simulink model "sensorExpoler_Lab1_1"  (R2026a)
settings: Solver=FixedStepAuto  StopTime=10  FixedStep=0.001
undefined symbols (not defined in the file or in its folder): Blocking, Non
libraries: amg_usbconverter_n_connect_lib x2
settings Model: Creator=pboon  LastModifiedBy=Kawpaan

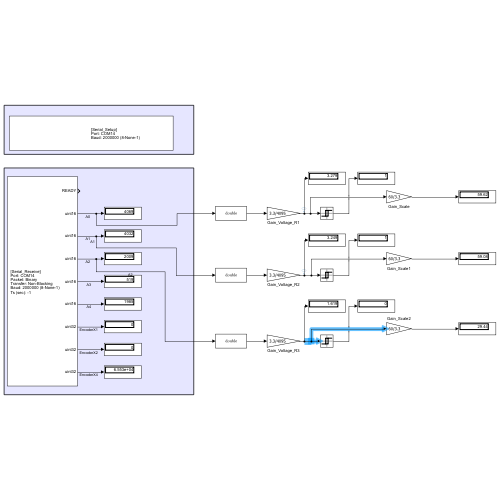
[thumbnail: Simulink's stored preview of the top-level diagram]
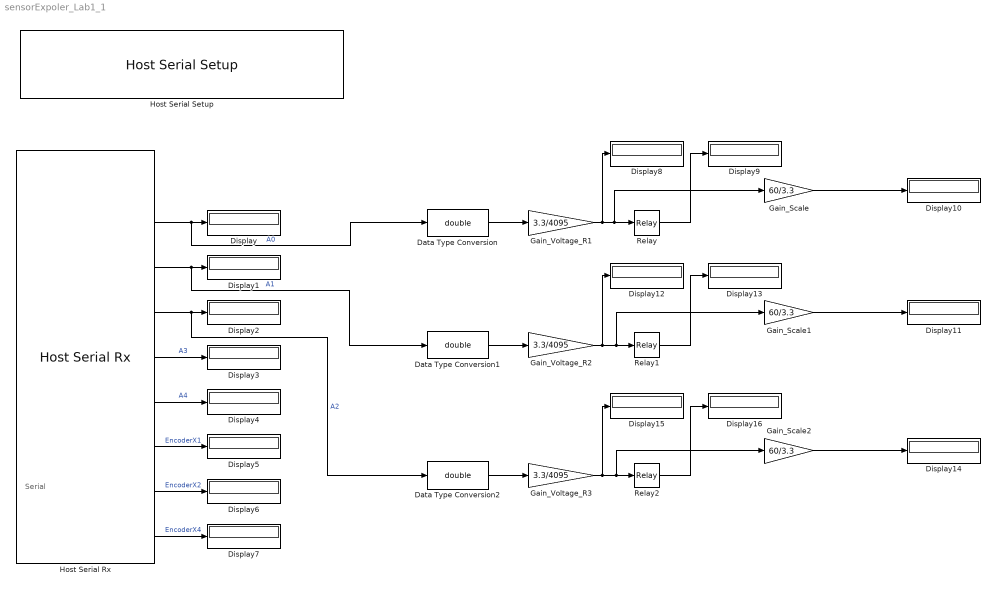
== system sensorExpoler_Lab1_1 ==
  note: Serial
  Data Type Conversion : DataTypeConversion  OutDataTypeStr=double  SaturateOnIntegerOverflow=off  RndMeth=Floor
  Data Type Conversion1 : DataTypeConversion  OutDataTypeStr=double  SaturateOnIntegerOverflow=off  RndMeth=Floor
  Data Type Conversion2 : DataTypeConversion  OutDataTypeStr=double  SaturateOnIntegerOverflow=off  RndMeth=Floor
  Display{,1..16} (17 alike) : Display
  Gain_Scale : Gain  Gain=60/3.3
  Gain_Scale1 : Gain  Gain=60/3.3
  Gain_Scale2 : Gain  Gain=60/3.3
  Gain_Voltage_R1 : Gain  Gain=3.3/4095
  Gain_Voltage_R2 : Gain  Gain=3.3/4095
  Gain_Voltage_R3 : Gain  Gain=3.3/4095
  Host Serial Rx : amg_usbconverter_n_connect_lib/Host Serial Rx  conf=rx  port=<auto>  baudrate=2000000  databits=8  parity=None  stopbit=1  flowcontrol=None  transfer=Non-Blocking  timeout=5  packetmode=Binary  enableinitialvalues=off  initialvalues=[]  binheader='25'  binterminator='4E 4E'  porttype_double=0  porttype_single=0  porttype_int8=0  porttype_uint8=0  porttype_int16=0  porttype_uint16=5  porttype_int32=0  porttype_uint32=3  asciiformat='%d,%f'  rx_asciiterminator="CRLF (0x0D 0x0A - \"\\r\\n\")"  tx_asciiterminator="CRLF (0x0D 0x0A - \"\\r\\n\")"  sampletime=0.001  enablecustomportlabel=off  cinputportlabel=0  coutputportlabel=A  portpinstr=0  blockid=HostSerialRx  inputporttype=[]  inputportwidth=[]  inputportlabel={}  outputporttype=[3 5 5 5 5 5 7 7 7]  outputportwidth=[1 1 1 1 1 1 1 1 1]  outputportlabel={'READY','uint16','uint16','uint16','uint16','uint16','uint32','uint32','uint32'}  compat=0  optionstring=[]  autoport='COM14'
  Host Serial Setup : amg_usbconverter_n_connect_lib/Host Serial Setup  conf=setup  port=<auto>  baudrate=2000000  databits=8  parity=None  stopbit=1  flowcontrol=None  transfer=Blocking  timeout=2  packetmode=Binary  initialvalues=[]  binheader='7E 7E'  binterminator='03 03'  porttype_double=0  porttype_single=1  porttype_int8=0  porttype_uint8=0  porttype_int16=0  porttype_uint16=0  porttype_int32=0  porttype_uint32=2  asciiformat='%d %u %x'  rx_asciiterminator="CRLF (0x0D 0x0A - \"\\r\\n\")"  tx_asciiterminator="CRLF (0x0D 0x0A - \"\\r\\n\")"  sampletime=-1  enablecustomportlabel=off  cinputportlabel=0  coutputportlabel=A  portpinstr=0  blockid=HostSerialSetup  inputporttype=[]  inputportwidth=[]  inputportlabel={}  outputporttype=[]  outputportwidth=[]  outputportlabel={}  compat=0  optionstring=[]  autoport='COM14'
  Relay : Relay  OnSwitchValue=2.2  OffSwitchValue=1.1
  Relay1 : Relay  OnSwitchValue=2.2  OffSwitchValue=1.1
  Relay2 : Relay  OnSwitchValue=2.2  OffSwitchValue=1.1
  wires:
  Host Serial Rx/2 -> Data Type Conversion/1, Display/1  "A0"
  Host Serial Rx/5 -> Display3/1  "A3"
  Host Serial Rx/6 -> Display4/1  "A4"
  Host Serial Rx/7 -> Display5/1  "EncoderX1"
  Host Serial Rx/8 -> Display6/1  "EncoderX2"
  Host Serial Rx/9 -> Display7/1  "EncoderX4"
  Data Type Conversion/1 -> Gain_Voltage_R1/1
  Gain_Voltage_R1/1 -> Display8/1, Gain_Scale/1, Relay/1
  Relay/1 -> Display9/1
  Gain_Scale/1 -> Display10/1
  Data Type Conversion1/1 -> Gain_Voltage_R2/1
  Relay1/1 -> Display13/1
  Gain_Scale1/1 -> Display11/1
  Gain_Voltage_R2/1 -> Display12/1, Gain_Scale1/1, Relay1/1
  Host Serial Rx/3 -> Data Type Conversion1/1, Display1/1  "A1"
  Data Type Conversion2/1 -> Gain_Voltage_R3/1
  Relay2/1 -> Display16/1
  Gain_Scale2/1 -> Display14/1
  Gain_Voltage_R3/1 -> Display15/1, Gain_Scale2/1, Relay2/1
  Host Serial Rx/4 -> Data Type Conversion2/1, Display2/1  "A2"
